simulink model "With-Attack"  (R2018b)
settings: Solver=VariableStepAuto  StartTime=0.0  StopTime=10  RelTol=1e-3
undefined symbols (not defined in the file or in its folder): sigbuilder_block
settings Model: Creator=lenovo  LastModifiedBy=lenovo

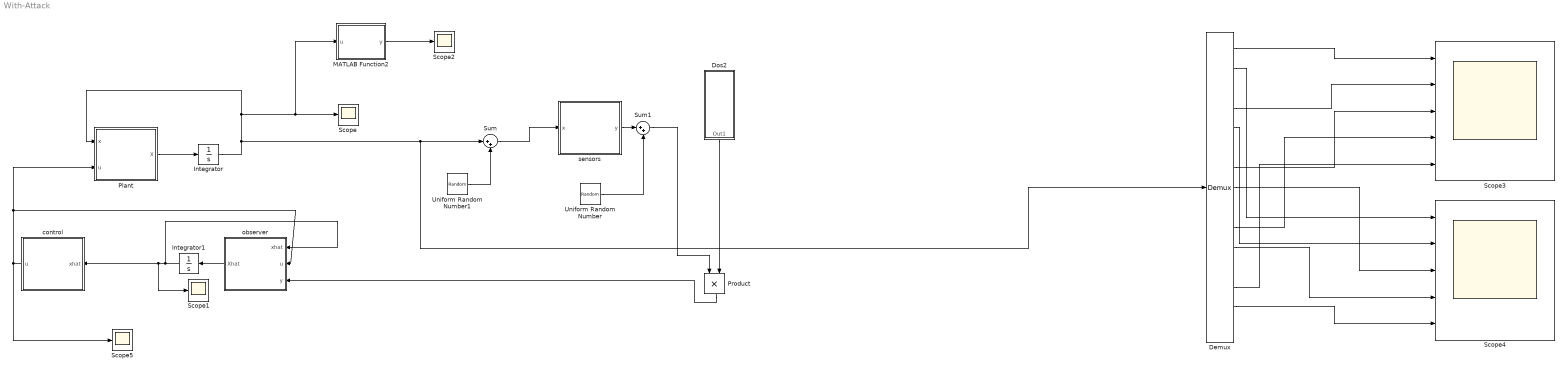
== system With-Attack ==
  Demux : Demux  Outputs=15
  Dos2 : Subsystem
  Integrator : Integrator  InitialCondition=10*[-7;-6;-5;-4;-3;-2;-1;0;1;2;3;4;5;6;7]
  Integrator1 : Integrator  InitialCondition=-10*[-7;-6;-5;-4;-3;-2;-1;0;1;2;3;4;5;6;7]
  MATLAB Function2 : MATLAB Function  TreatAsAtomicUnit=on
  Plant : MATLAB Function  TreatAsAtomicUnit=on
  Product : Product
  Scope{,1..2,5} (4 alike) : Scope
  Scope3 : Scope  NumInputPorts=5
  Scope4 : Scope  NumInputPorts=5
  Sum : Sum  Inputs=|++
  Sum1 : Sum  Inputs=|++
  Uniform Random Number : UniformRandomNumber  Minimum=-0.01  Maximum=0.01  SampleTime=0.1
  Uniform Random Number1 : UniformRandomNumber  Minimum=-0.01  Maximum=0.01  SampleTime=0.1
  control : MATLAB Function  TreatAsAtomicUnit=on
  observer : MATLAB Function  TreatAsAtomicUnit=on
  sensors : MATLAB Function  TreatAsAtomicUnit=on
  wires:
  Dos2/1(Out1) -> Product/2
  sensors/1(y) -> Sum1/1
  Uniform Random Number/1 -> Sum1/2
  Plant/1(X) -> Integrator/1
  Integrator1/1 -> Scope1/1, control/1(xhat), observer/1(xhat)
  Uniform Random Number1/1 -> Sum/2
  Sum/1 -> sensors/1(x)
  control/1(u) -> Plant/2(u), observer/2(u), Scope5/1
  MATLAB Function2/1(y) -> Scope2/1
  observer/1(Xhat) -> Integrator1/1
  Sum1/1 -> Product/1
  Product/1 -> observer/3(y)
  Demux/10 -> Scope3/4
  Integrator/1 -> Demux/1, Sum/1, Plant/1(x), MATLAB Function2/1(u), Scope/1
  Demux/1 -> Scope3/1
  Demux/2 -> Scope4/1
  Demux/13 -> Scope3/5
  Demux/7 -> Scope3/3
  Demux/8 -> Scope4/3
  Demux/5 -> Scope4/2
  Demux/4 -> Scope3/2
  Demux/11 -> Scope4/4
  Demux/14 -> Scope4/5

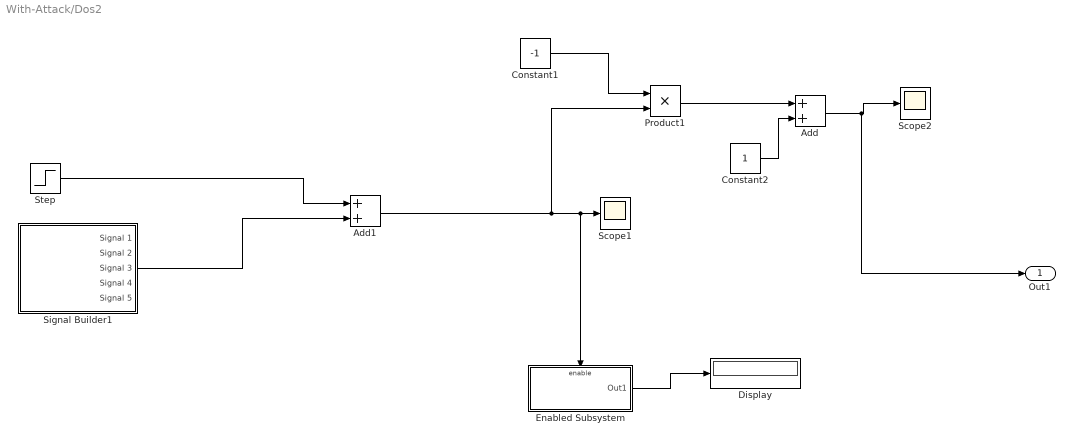
== system With-Attack/Dos2 ==
  Add : Sum
  Add1 : Sum
  Constant1 : Constant  Value=-1
  Constant2 : Constant
  Display : Display
  Enabled Subsystem : Subsystem  TreatAsAtomicUnit=on
  Product1 : Product
  Scope1 : Scope
  Scope2 : Scope
  Signal Builder1 : Subsystem  Tag=STV Subsys  LoadFcn=sigbuilder_block('load');  StartFcn=sigbuilder_block('start');  StopFcn=sigbuilder_block('stop');  ClipboardFcn=sigbuilder_block('clipboard');  mask(Sigbuilder block){tuvar=[0:10]}
      mask help: Simulink:masks:SigbuilderBlock_MD
      mask init:
      | if ~strcmp(get_param(bdroot(gcbh),'SimulationStatus'),'stopped') tuvar = sigbuilder_block('maskInit'); end
      settings: CopyFcn=sigbuilder_block('copy');  DeleteFcn=sigbuilder_block('delete');  ModelCloseFcn=sigbuilder_block('modelClose');  PreSaveFcn=sigbuilder_block('preSave');  PauseFcn=sigbuilder_block('pause');  ContinueFcn=sigbuilder_block('continue');  NameChangeFcn=sigbuilder_block('namechange');  OpenFcn=sigbuilder_block('open',[5.4 30 1141.2 522.6 ]);  CloseFcn=sigbuilder_block('close');
      mask Display: plot(0, 0, 100, 100,[2, 2, 32, 32, 2], [68, 8, 8, 68, 68],[32, 2], [38, 38], [32, 19, 2],[53, 60, 44], [32, 17, 17, 2],[16, 16, 31, 31]);txt = getActiveGroup(gcbh);text(2, 100, txt,'verticalAlignment', 'top');
  Step : Step  After=-1  SampleTime=10
  Out1 : Outport
  wires:
  Enabled Subsystem/1(Out1) -> Display/1
  Constant1/1 -> Product1/1
  Product1/1 -> Add/1
  Constant2/1 -> Add/2
  Add/1 -> Out1/1, Scope2/1
  Step/1 -> Add1/1
  Add1/1 -> Product1/2, Enabled Subsystem/Enable, Scope1/1
  Signal Builder1/3(Signal 3) -> Add1/2

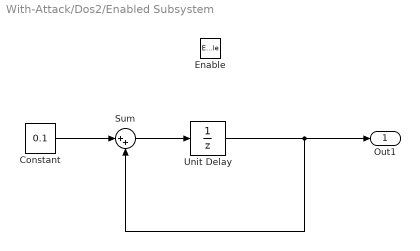
== system With-Attack/Dos2/Enabled Subsystem ==
  Enable : EnablePort
  Constant : Constant  Value=0.1
  Sum : Sum  Inputs=|++
  Unit Delay : UnitDelay  SampleTime=-1
  Out1 : Outport
  wires:
  Unit Delay/1 -> Out1/1, Sum/2
  Constant/1 -> Sum/1
  Sum/1 -> Unit Delay/1

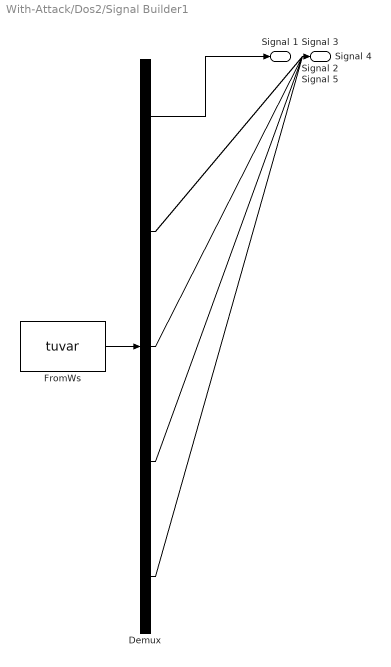
== system With-Attack/Dos2/Signal Builder1 ==
  Demux : Demux  Tag=STV Demux  Outputs=5
  FromWs : FromWorkspace  Tag=STV FromWs  VariableName=tuvar  SampleTime=0
      SigBuilderData=|
      | common.afterFinalStr = 'Extrapolate'
      | common.sampleTime = 0
      | dataSet.timeRange = [0 10]
      | dataSet.name = 'Group 1'
      | sbobj.Groups.Name = 'Group 1'
      | sbobj.Groups.Signals(1).Name = 'Signal 1'
      | sbobj.Groups.Signals(1).XData = [0 4 4 6 6 10]
      | sbobj.Groups.Signals(1).YData = [0 0 1 1 0 0]
      | sbobj.Groups.Signals(2).Name = 'Signal 2'
      | sbobj.Groups.Signals(2).XData = [0 0.125 0.125 0.25 0.25 0.375 0.375 0.5 0.5 0.625 0.625 0.75 0.75 0.875 0.875 1 1 1.125 1.125 1.25 1.25 1.375 1.375 1.5 1.5 1.625 1.625 1.75 1.75 1.875 1.875 2 2 2.125 2.125 2.25 2.25 2.375 2.375 2.5 2.5 2.625 2.625 2.75 2.75 2.875 2.875 3 3 3.125 3.125 3.25 3.25 3.375 3.375 3.5 3.5 3.625 3.625 3.75 3.75 3.875 3.875 4 4 4.125 4.125 4.25 4.25 4.375 4.375 4.5 4.5 4.625 4.625 4.75 4.75 4.875 4.875 5 5 5.125 5.125 5.25 5.25 5.375 5.375 5.5 5.5 5.625 5.625 5.75 5.75 5.875 5.875 6 6 6.125 6.125 6.25 6.25 6.375 6.375 6.5 6.5 6.625 6.625 6.75 6.75 6.875 6.875 7 7 7.125 7.125 7.25 7.25 7.375 7.375 7.5 7.5 7.625 7.625 7.75 7.75 7.875 7.875 8 8 8.125 8.125 8.25 8.25 8.375 8.375 8.5 8.5 8.625 8.625 8.75 8.75 8.875 8.875 9 9 9.125 9.125 9.25 9.25 9.375 9.375 9.5 9.5 9.625 9.625 9.75 9.75 9.875 9.875 10]
      | sbobj.Groups.Signals(2).YData = [1 1 -1 -1 1 1 -1 -1 1 1 -1 -1 1 1 -1 -1 1 1 -1 -1 1 1 -1 -1 1 1 -1 -1 1 1 -1 -1 1 1 -1 -1 1 1 -1 -1 1 1 -1 -1 1 1 -1 -1 1 1 -1 -1 1 1 -1 -1 1 1 -1 -1 1 1 -1 -1 1 1 -1 -1 1 1 -1 -1 1 1 -1 -1 1 1 -1 -1 1 1 -1 -1 1 1 -1 -1 1 1 -1 -1 1 1 -1 -1 1 1 -1 -1 1 1 -1 -1 1 1 -1 -1 1 1 -1 -1 1 1 -1 -1 1 1 -1 -1 1 1 -1 -1 1 1 -1 -1 1 1 -1 -1 1 1 -1 -1 1 1 -1 -1 1 1 -1 -1 1 1 -1 -1 1 1 -1 -1 1 1 -1 -1 1 1 -1 -1]
      | sbobj.Groups.Signals(3).Name = 'Signal 3'
      | sbobj.Groups.Signals(3).XData = [0 0.16 0.333333333333 0.4 0.4 0.46 0.46 0.833333333333 1 1.005 1.005 1.3 1.3 1.8 1.8 1.9 1.9 2.4 2.4 2.55 2.55 2.625 2.785 2.83333333333 3 3.2 3.2 3.4 3.4 3.5 3.66666666667 3.83333333333 4 4 4.17 4.17 4.33333333333 4.5 4.8 4.8 4.85 4.85 5 5.16666666667 5.33333333333 5.33333333333 5.5 5.5 5.66666666667 5.83333333333 5.83333333333 6 6 6.16666666667 6.33333333333 6.5 6.5 6.66666666667 6.66666666667 6.83333333333 7 7 7.16666666667 7.16666666667 7.33333333333 7.5 7.66666666667 7.83333333333 7.83333333333 8 8 8.16666666667 8.33333333333 8.5 8.5 8.66666666667 8.66666666667 8.83333333333 9 9.16666666667 9.33333333333 9.33333333333 9.5 9.5 9.66666666667 9.83333333333 10]
      | sbobj.Groups.Signals(3).YData = [1 1 1 1 0 0 1 1 1 1 0 0 1 1 0 0 1 1 0 0 1 1 1 1 1 1 0 0 1 1 1 1 1 0 0 1 1 1 1 0 0 1 1 1 1 0 0 1 1 1 0 0 1 1 1 1 0 0 1 1 1 0.005 0.005 1 1 1 1 1 0 0 1 1 1 1 0 0 1 1 1 1 1 0 0 1 1 1 1]
      | sbobj.Groups.Signals(4).Name = 'Signal 4'
      | sbobj.Groups.Signals(4).XData = [0 5 5 10]
      | sbobj.Groups.Signals(4).YData = [0 0 1 1]
      | sbobj.Groups.Signals(5).Name = 'Signal 5'
      | sbobj.Groups.Signals(5).XData = [0 0.45 0.45 0.5 0.5 0.95 0.95 1 1 1.45 1.45 1.5 1.5 1.95 1.95 2 2 2.45 2.45 2.5 2.5 2.95 2.95 3 3 3.45 3.45 3.5 3.5 3.95 3.95 4 4 4.45 4.45 4.5 4.5 4.95 4.95 5 5 5.45 5.45 5.5 5.5 5.95 5.95 6 6 6.45 6.45 6.5 6.5 6.95 6.95 7 7 7.45 7.45 7.5 7.5 7.95 7.95 8 8 8.45 8.45 8.5 8.5 8.95 8.95 9 9 9.45 9.45 9.5 9.5 9.95 9.95 10]
      | sbobj.Groups.Signals(5).YData = [1 1 0 0 1 1 0 0 1 1 0 0 1 1 0 0 1 1 0 0 1 1 0 0 1 1 0 0 1 1 0 0 1 1 0 0 1 1 0 0 1 1 0 0 1 1 0 0 1 1 0 0 1 1 0 0 1 1 0 0 1 1 0 0 1 1 0 0 1 1 0 0 1 1 0 0 0.995 0.995 0 0]
  Signal 1 : Outport  Tag=STV Outport
  Signal 2 : Outport  Tag=STV Outport  Port=2
  Signal 3 : Outport  Tag=STV Outport  Port=3
  Signal 4 : Outport  Tag=STV Outport  Port=4
  Signal 5 : Outport  Tag=STV Outport  Port=5
  wires:
  Demux/1 -> Signal 1/1
  FromWs/1 -> Demux/1
  Demux/2 -> Signal 2/1
  Demux/3 -> Signal 3/1
  Demux/4 -> Signal 4/1
  Demux/5 -> Signal 5/1

== matlab function With-Attack/control ==
  data: xhat input; u output
function u = fcn(xhat)
A=[ 1.049     0.03183    -0.02926
     0.01347       1.023  -0.0001932
  -0.0007729     -0.1155      0.9048];
B=[0.2026  6.946e-05
   -0.1504     0.1012
  0.008724    0.08931 ];
L=[ 1 0 0 0 -1; -1 1 0 0 0; -1 0 1 0 0; 0 -1 0 1 0; 0 -1 -1 -1 3];
A0=kron(eye(5),A);
B0=kron(eye(5),B);
z=kron(L,eye(3));
Q=z'*eye(15)*z;

q1=[1.9115   -1.1429    0.4148    0.0000    0.0000   -0.0000    0.0000    0.0000   -0.0000
    3.0186    4.4625   -0.5557   -0.0000   -0.0000    0.0000   -0.0000   -0.0000    0.0000
    0.0000    0.0000   -0.0000    1.9115   -1.1429    0.4148    0.0000    0.0000   -0.0000
   -0.0000   -0.0000    0.0000    3.0186    4.4625   -0.5557   -0.0000   -0.0000    0.0000
    0.0000    0.0000   -0.0000    0.0000    0.0000   -0.0000    1.9115   -1.1429    0.4148
   -0.0000   -0.0000    0.0000   -0.0000   -0.0000    0.0000    3.0186    4.4625   -0.5557
    0.0000    0.0000   -0.0000    0.0000    0.0000    0.0000    0.0000    0.0000   -0.0000
    0.0000    0.0000   -0.0000    0.0000    0.0000   -0.0000   -0.0000   -0.0000    0.0000
    0.0000    0.0000   -0.0000   -0.0000   -0.0000    0.0000   -0.0000   -0.0000    0.0000
    0.0000    0.0000   -0.0000    0.0000    0.0000   -0.0000    0.0000    0.0000   -0.0000
];
q2=[-0.0000   -0.0000    0.0000   -0.0000   -0.0000    0.0000
    0.0000    0.0000   -0.0000    0.0000    0.0000    0.0000
    0.0000    0.0000   -0.0000   -0.0000   -0.0000    0.0000
   -0.0000   -0.0000    0.0000    0.0000    0.0000   -0.0000
    0.0000    0.0000   -0.0000    0.0000    0.0000   -0.0000
   -0.0000   -0.0000    0.0000    0.0000    0.0000   -0.0000
    1.9115   -1.1429    0.4148   -0.0000   -0.0000    0.0000
    3.0186    4.4625   -0.5557   -0.0000   -0.0000    0.0000
    0.0000    0.0000   -0.0000    1.9115   -1.1429    0.4148
   -0.0000   -0.0000    0.0000    3.0186    4.4625   -0.5557
];
% K=[    1.9115   -1.1429    0.4148
%     3.0186    4.4625   -0.5557];
K=[q1 q2];
u=-K*xhat;

== matlab function With-Attack/Plant ==
  data: x input; X output; u input
function X = fcn(x,u)
A=[.48 .29 -.3;.13 .23 0;0 -1.2 -1];
B=[2 0;-1.5 1; 0 1];
A0=kron(eye(5),A);
B0=kron(eye(5),B);
X =A0*x+B0*u;

== matlab function With-Attack/sensors ==
  data: x input; y output
function y = fcn(x)
C=eye(3);
C0=kron(eye(5),C);
y=C0*x;

== matlab function With-Attack/observer ==
  data: xhat input; u input; Xhat output; y input
function Xhat = fcn(xhat,u,y)
A=[.48 .29 -.3;.13 .23 0;0 -1.2 -1];
B=[2 0;-1.5 1; 0 1];
C=eye(3);
G=[ 5.0468    1.5160   -0.5215
    1.5160    1.8633   -0.6870
   -0.5215   -0.6870    1.1919];
C0=kron(eye(5),C);
A0=kron(eye(5),A);
B0=kron(eye(5),B);
G0=kron(eye(5),G);
yhat=C0*xhat;
Xhat=A0*xhat+B0*u+G0*(y-yhat);

== matlab function With-Attack/MATLAB Function2 ==
  data: u input; y output
function y = fcn(u)
y=norm(u);
